simulink model "Edge_detector"  (Simulink 7.6)
settings: Solver=FixedStepDiscrete  SolverMode=SingleTasking  StartTime=0.0  StopTime=307201.0  RelTol=1e-3
InitFcn:
  | ed_in_script
  | %% DSPBuilder Start
  | alt_dspbuilder_update_model(bdroot)
  | %% DSPBuilder End
StopFcn:
  | ed_out_script
libraries: allblocks_alteradspbuilder2 x45
settings Model: Creator=lkong  LastModifiedBy=akarapet
settings DataIOCC: SignalLoggingName=sigsOut
settings OptimizationCC: InlineInvariantSignals=on  InitFltsAndDblsToZero=on
settings DebuggingCC: SaveWithParameterizedLinksMsg=none  SignalResolutionControl=TryResolveAllWithWarning  SolverPrmCheckMsg=none  MultiTaskDSMMsg=warning  MultiTaskCondExecSysMsg=none  StrictBusMsg=None
settings HardwareCC: TargetUnknown=on
settings RTWCC: IncludeERTFirstTime=on
settings GRTTargetCC: TargetFcnLib=ansi_tfl_tmw.mat

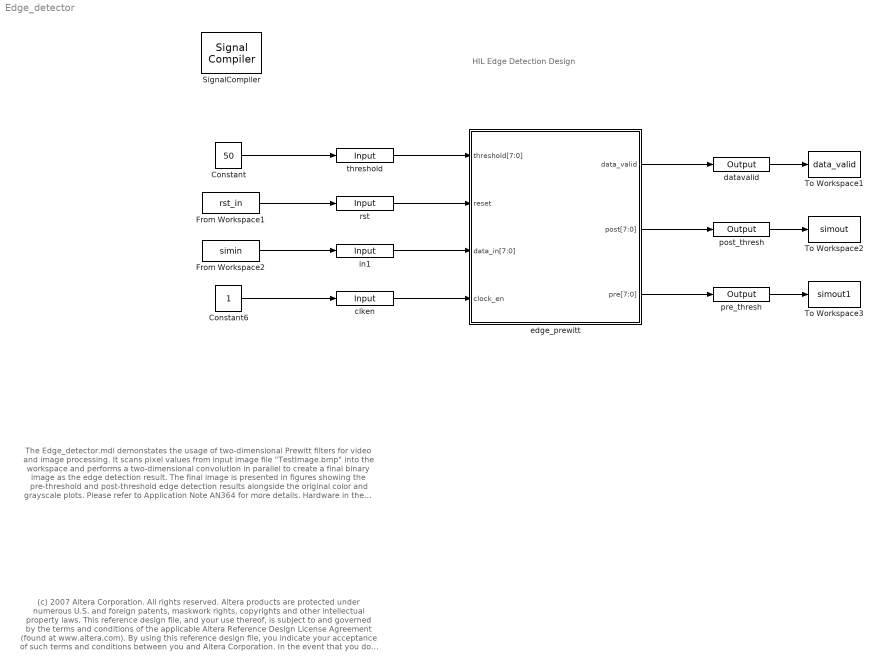
== system Edge_detector ==
  note: HIL Edge Detection Design
  note: The Edge_detector.mdl demonstates the usage of two-dimensional Prewitt filters for video and image processing.
      | It scans pixel values from input image file "TestImage.bmp" into the workspace and performs a two-dimensional
      | convolution in parallel to create a final binary image as the edge detection result.
      |
      | The final image is presented in figures showing the pre-threshold and post-threshold edge detection results
      | alongside the original color and grayscale plots.
      |
      | Please refer to Application Note AN364 for more details.
      |
      | Hardware in the Loop (HIL) is used to speed-up simulation as well as to verify the design in hardware.
  note: (c) 2007 Altera Corporation. All rights reserved.  Altera products are protected under numerous U.S. and foreign patents, maskwork rights, copyrights and other intellectual property laws.
      | This reference design file, and your use thereof, is subject to and governed by the terms and conditions of the applicable Altera Reference Design License Agreement (found at www.altera.com).
      | By using this reference design file, you indicate your acceptance of such terms and conditions between you and Altera Corporation.
      | In the event that you do not agree with such terms and conditions, you may not use the reference design file and please promptly destroy any copies you have made.
      | This reference design file being provided on an "as-is" basis and as an accommodation and therefore all warranties, representations or guarantees of any kind (whether express, implied or statutory)
      | including, without limitation, warranties of merchantability, non-infringement, or fitness for a particular purpose, are specifically disclaimed.
      | By making this reference design file available, Altera expressly does not recommend, suggest or require that this reference design file be used in combination with any other product not provided by Altera
  Constant : Constant  Value=50
  Constant6 : Constant
  From Workspace1 : FromWorkspace  VariableName=rst_in  SampleTime=1
  From Workspace2 : FromWorkspace  VariableName=simin  SampleTime=1
  SignalCompiler : allblocks_alteradspbuilder2/Signal Compiler  DeviceFamily=Cyclone III  DeviceName=EP3C120F780C7  EnableSignalTap=off  SignalTapDepth=1024  UseBoardBlock=off  StpUseDefaultClock=on  StpClock=Clock  ExportDir=/data/akarapet/qshell_linux64_test/p4/dsp_builder/dsp_builder2/Documentation/DesignExamples/Tutorials/HIL/EdgeDetection
  To Workspace1 : ToWorkspace  VariableName=data_valid  SaveFormat=Array
  To Workspace2 : ToWorkspace  VariableName=simout  SaveFormat=Array
  To Workspace3 : ToWorkspace  VariableName=simout1  SaveFormat=Array
  clken : allblocks_alteradspbuilder2/Input  iofile=/data/akarapet/qshell_linux64_test/p4/dsp_builder/dsp_builder2/Documentation/DesignExamples/Tutorials/HIL/EdgeDetection/tb_Edge_detector/Edge%5Fdetector_clken.salt  BusType=Single Bit  bwl=1  bwr=0  SpecifyClock=off  PORTTYPE=Input  externalType=Inferred  allowFloatingPointOverride=on  logOutputs=off
  datavalid : allblocks_alteradspbuilder2/Output  iofile=/data/akarapet/qshell_linux64_test/p4/dsp_builder/dsp_builder2/Documentation/DesignExamples/Tutorials/HIL/EdgeDetection/tb_Edge_detector/Edge%5Fdetector_datavalid.capture  BusType=Single Bit  bwl=1  bwr=0  externalType=Inferred  PORTTYPE=Output  allowFloatingPointOverride=on  logOutputs=off
  edge_prewitt : Subsystem
      mask Type: SubSystem AlteraBlockSet
  in1 : allblocks_alteradspbuilder2/Input  iofile=/data/akarapet/qshell_linux64_test/p4/dsp_builder/dsp_builder2/Documentation/DesignExamples/Tutorials/HIL/EdgeDetection/tb_Edge_detector/Edge%5Fdetector_in1.salt  BusType=Unsigned Integer  bwl=8  bwr=0  SpecifyClock=off  PORTTYPE=Input  externalType=Inferred  allowFloatingPointOverride=on  logOutputs=off
  post_thresh : allblocks_alteradspbuilder2/Output  iofile=/data/akarapet/qshell_linux64_test/p4/dsp_builder/dsp_builder2/Documentation/DesignExamples/Tutorials/HIL/EdgeDetection/tb_Edge_detector/Edge%5Fdetector_post%5Fthresh.capture  BusType=Unsigned Integer  bwl=8  bwr=0  externalType=Inferred  PORTTYPE=Output  allowFloatingPointOverride=on  logOutputs=off
  pre_thresh : allblocks_alteradspbuilder2/Output  iofile=/data/akarapet/qshell_linux64_test/p4/dsp_builder/dsp_builder2/Documentation/DesignExamples/Tutorials/HIL/EdgeDetection/tb_Edge_detector/Edge%5Fdetector_pre%5Fthresh.capture  BusType=Unsigned Integer  bwl=8  bwr=0  externalType=Inferred  PORTTYPE=Output  allowFloatingPointOverride=on  logOutputs=off
  rst : allblocks_alteradspbuilder2/Input  iofile=/data/akarapet/qshell_linux64_test/p4/dsp_builder/dsp_builder2/Documentation/DesignExamples/Tutorials/HIL/EdgeDetection/tb_Edge_detector/Edge%5Fdetector_rst.salt  BusType=Single Bit  bwl=1  bwr=0  SpecifyClock=off  PORTTYPE=Input  externalType=Inferred  allowFloatingPointOverride=on  logOutputs=off
  threshold : allblocks_alteradspbuilder2/Input  iofile=/data/akarapet/qshell_linux64_test/p4/dsp_builder/dsp_builder2/Documentation/DesignExamples/Tutorials/HIL/EdgeDetection/tb_Edge_detector/Edge%5Fdetector_threshold.salt  BusType=Unsigned Integer  bwl=8  bwr=0  SpecifyClock=off  PORTTYPE=Input  externalType=Inferred  allowFloatingPointOverride=on  logOutputs=off
  wires:
  Constant6/1 -> clken/1
  Constant/1 -> threshold/1
  From Workspace1/1 -> rst/1
  clken/1 -> edge_prewitt/4(clock_en)
  From Workspace2/1 -> in1/1
  in1/1 -> edge_prewitt/3(data_in[7:0])
  rst/1 -> edge_prewitt/2(reset)
  threshold/1 -> edge_prewitt/1(threshold[7:0])
  datavalid/1 -> To Workspace1/1
  edge_prewitt/2(post[7:0]) -> post_thresh/1
  edge_prewitt/1(data_valid) -> datavalid/1
  pre_thresh/1 -> To Workspace3/1
  post_thresh/1 -> To Workspace2/1
  edge_prewitt/3(pre[7:0]) -> pre_thresh/1

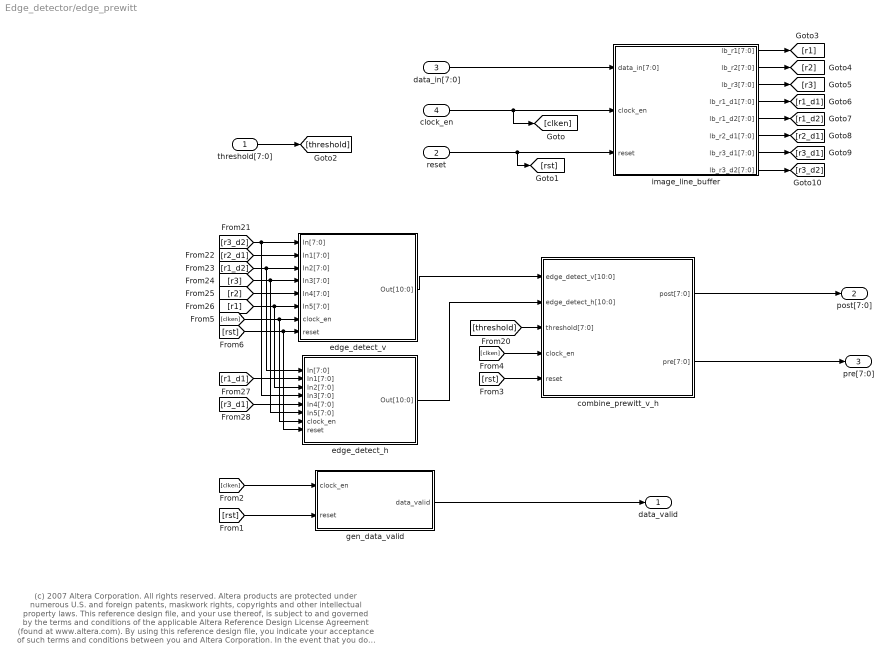
== system Edge_detector/edge_prewitt ==
  note: (c) 2007 Altera Corporation. All rights reserved.  Altera products are protected under numerous U.S. and foreign patents, maskwork rights, copyrights and other intellectual property laws.
      | This reference design file, and your use thereof, is subject to and governed by the terms and conditions of the applicable Altera Reference Design License Agreement (found at www.altera.com).
      | By using this reference design file, you indicate your acceptance of such terms and conditions between you and Altera Corporation.
      | In the event that you do not agree with such terms and conditions, you may not use the reference design file and please promptly destroy any copies you have made.
      | This reference design file being provided on an "as-is" basis and as an accommodation and therefore all warranties, representations or guarantees of any kind (whether express, implied or statutory)
      | including, without limitation, warranties of merchantability, non-infringement, or fitness for a particular purpose, are specifically disclaimed.
      | By making this reference design file available, Altera expressly does not recommend, suggest or require that this reference design file be used in combination with any other product not provided by Altera
  threshold[7:0] : Inport
  reset : Inport  Port=2
  data_in[7:0] : Inport  Port=3
  clock_en : Inport  Port=4
  combine_prewitt_v_h : Subsystem
      mask Type: SubSystem AlteraBlockSet
  edge_detect_h : Subsystem  AncestorBlock=ALTELINK/AltLab/HDL SubSystem
      mask Type: SubSystem AlteraBlockSet
  edge_detect_v : Subsystem  AncestorBlock=ALTELINK/AltLab/HDL SubSystem
      mask Type: SubSystem AlteraBlockSet
  gen_data_valid : Subsystem
      mask Type: SubSystem AlteraBlockSet
  image_line_buffer : Subsystem
      mask Type: SubSystem AlteraBlockSet
  data_valid : Outport
  post[7:0] : Outport  Port=2
  pre[7:0] : Outport  Port=3
  wires:
  edge_detect_v/1(Out[10:0]) -> combine_prewitt_v_h/1(edge_detect_v[10:0])
  edge_detect_h/1(Out[10:0]) -> combine_prewitt_v_h/2(edge_detect_h[10:0])
  [r3_d2] -> edge_detect_v/1(In[7:0]), edge_detect_h/4(In3[7:0])
  [r2_d1] -> edge_detect_v/2(In1[7:0])
  [r1_d2] -> edge_detect_v/3(In2[7:0]), edge_detect_h/1(In[7:0])
  [r3] -> edge_detect_v/4(In3[7:0]), edge_detect_h/6(In5[7:0])
  [r2] -> edge_detect_v/5(In4[7:0])
  [r1] -> edge_detect_v/6(In5[7:0]), edge_detect_h/3(In2[7:0])
  [r1_d1] -> edge_detect_h/2(In1[7:0])
  [r3_d1] -> edge_detect_h/5(In4[7:0])
  gen_data_valid/1(data_valid) -> data_valid/1
  image_line_buffer/1(lb_r1[7:0]) -> [r1]
  image_line_buffer/2(lb_r2[7:0]) -> [r2]
  image_line_buffer/3(lb_r3[7:0]) -> [r3]
  image_line_buffer/4(lb_r1_d1[7:0]) -> [r1_d1]
  image_line_buffer/5(lb_r1_d2[7:0]) -> [r1_d2]
  image_line_buffer/6(lb_r2_d1[7:0]) -> [r2_d1]
  image_line_buffer/7(lb_r3_d1[7:0]) -> [r3_d1]
  image_line_buffer/8(lb_r3_d2[7:0]) -> [r3_d2]
  [clken] -> gen_data_valid/1(clock_en)
  [rst] -> gen_data_valid/2(reset)
  [threshold] -> combine_prewitt_v_h/3(threshold[7:0])
  [clken] -> combine_prewitt_v_h/4(clock_en)
  [rst] -> combine_prewitt_v_h/5(reset)
  combine_prewitt_v_h/2(pre[7:0]) -> pre[7:0]/1
  combine_prewitt_v_h/1(post[7:0]) -> post[7:0]/1
  reset/1 -> image_line_buffer/3(reset), [rst]
  data_in[7:0]/1 -> image_line_buffer/1(data_in[7:0])
  clock_en/1 -> image_line_buffer/2(clock_en), [clken]
  [clken] -> edge_detect_v/7(clock_en), edge_detect_h/7(clock_en)
  [rst] -> edge_detect_v/8(reset), edge_detect_h/8(reset)
  threshold[7:0]/1 -> [threshold]

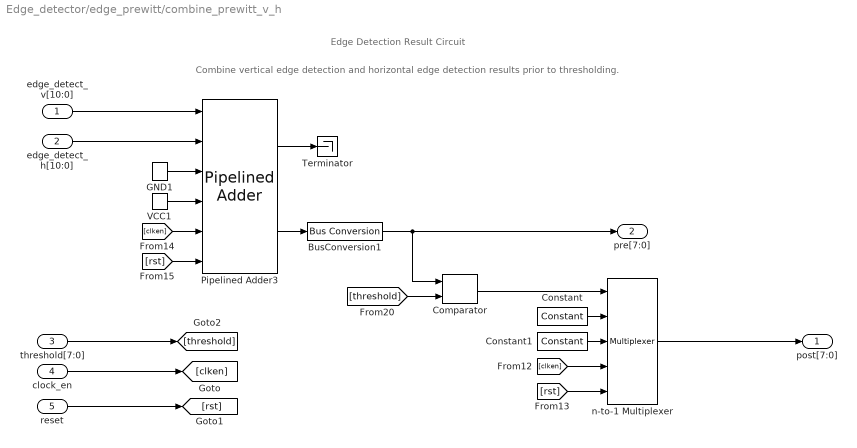
== system Edge_detector/edge_prewitt/combine_prewitt_v_h ==
  note: Combine vertical edge detection and horizontal edge detection results prior to thresholding.
  note: Edge Detection Result Circuit
  edge_detect_v[10:0] : Inport
  edge_detect_h[10:0] : Inport  Port=2
  threshold[7:0] : Inport  Port=3
  clock_en : Inport  Port=4
  reset : Inport  Port=5
  BusConversion1 : allblocks_alteradspbuilder2/Bus Conversion  BusType=Unsigned Integer  ibwl=11  ibwr=0  bwl=8  bwr=0  bitToConnectToOutputLSB=0  round=off  saturate=on  pipeline_display=0
  Comparator : allblocks_alteradspbuilder2/Comparator  direction=a < b  pipeline_display=0  allowFloatingPointOverride=on  logOutputs=off  logFile=/data/akarapet/qshell_linux64_test/p4/dsp_builder/dsp_builder2/Documentation/DesignExamples/Tutorials/HIL/EdgeDetection/tb_Edge_detector/Edge%5Fdetector_edge%5Fprewitt_combine%5Fprewitt%5Fv%5Fh_Comparator.fixedpointlog
  Constant : allblocks_alteradspbuilder2/Constant  mask_cst=255  BusType=Unsigned Integer  bwl=8  bwr=0  roundMode=Truncate  satMode=Wrap  SpecifyClock=off  allowFloatingPointOverride=on  logOutputs=off  logFile=/data/akarapet/qshell_linux64_test/p4/dsp_builder/dsp_builder2/Documentation/DesignExamples/Tutorials/HIL/EdgeDetection/tb_Edge_detector/Edge%5Fdetector_edge%5Fprewitt_combine%5Fprewitt%5Fv%5Fh_Constant.fixedpointlog
  Constant1 : allblocks_alteradspbuilder2/Constant  mask_cst=0  BusType=Unsigned Integer  bwl=8  bwr=0  roundMode=Truncate  satMode=Wrap  SpecifyClock=off  allowFloatingPointOverride=on  logOutputs=off  logFile=/data/akarapet/qshell_linux64_test/p4/dsp_builder/dsp_builder2/Documentation/DesignExamples/Tutorials/HIL/EdgeDetection/tb_Edge_detector/Edge%5Fdetector_edge%5Fprewitt_combine%5Fprewitt%5Fv%5Fh_Constant1.fixedpointlog
  GND1 : allblocks_alteradspbuilder2/GND  SpecifyClock=off
  Pipelined Adder3 : allblocks_alteradspbuilder2/Pipelined Adder  BusType=Unsigned Integer  bwl=11  bwr=0  pipeline=1  pipeline_display=1  AddSubDirection=ADD  use_cin=on  use_ovl=on  use_addsub=on  use_ena=on  use_aclr=on  or_aclr_inputs=on
  Terminator : Terminator
  VCC1 : allblocks_alteradspbuilder2/VCC  SpecifyClock=off
  n-to-1 Multiplexer : allblocks_alteradspbuilder2/Multiplexer  numInputs=2  pipeline=1  oneHot=off  pipeline_display=1  use_ena=on  use_aclr=on  allowFloatingPointOverride=on  logOutputs=off  logFile=/data/akarapet/qshell_linux64_test/p4/dsp_builder/dsp_builder2/Documentation/DesignExamples/Tutorials/HIL/EdgeDetection/tb_Edge_detector/Edge%5Fdetector_edge%5Fprewitt_combine%5Fprewitt%5Fv%5Fh_n-to-1+Multiplexer.fixedpointlog
  post[7:0] : Outport
  pre[7:0] : Outport  Port=2
  wires:
  Comparator/1 -> n-to-1 Multiplexer/1
  Constant/1 -> n-to-1 Multiplexer/2
  Constant1/1 -> n-to-1 Multiplexer/3
  BusConversion1/1 -> Comparator/1, pre[7:0]/1
  [clken] -> n-to-1 Multiplexer/4
  [rst] -> n-to-1 Multiplexer/5
  Pipelined Adder3/2 -> BusConversion1/1
  GND1/1 -> Pipelined Adder3/3
  VCC1/1 -> Pipelined Adder3/4
  [clken] -> Pipelined Adder3/5
  [rst] -> Pipelined Adder3/6
  edge_detect_v[10:0]/1 -> Pipelined Adder3/1
  edge_detect_h[10:0]/1 -> Pipelined Adder3/2
  threshold[7:0]/1 -> [threshold]
  reset/1 -> [rst]
  n-to-1 Multiplexer/1 -> post[7:0]/1
  clock_en/1 -> [clken]
  [threshold] -> Comparator/2
  Pipelined Adder3/1 -> Terminator/1

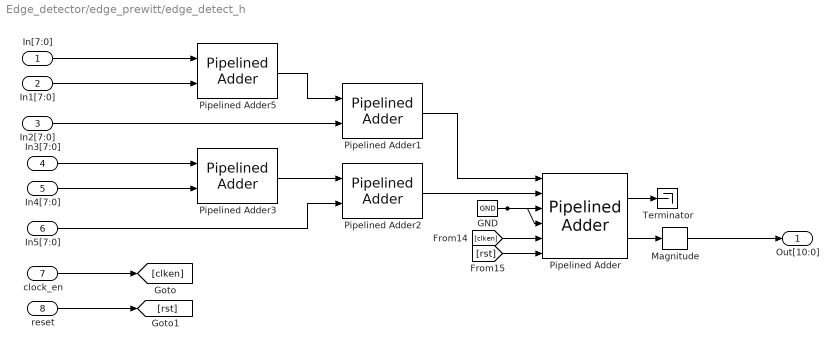
== system Edge_detector/edge_prewitt/edge_detect_h ==
  In[7:0] : Inport
  In1[7:0] : Inport  Port=2
  In2[7:0] : Inport  Port=3
  In3[7:0] : Inport  Port=4
  In4[7:0] : Inport  Port=5
  In5[7:0] : Inport  Port=6
  clock_en : Inport  Port=7
  reset : Inport  Port=8
  GND : allblocks_alteradspbuilder2/GND  SpecifyClock=off
  Magnitude : allblocks_alteradspbuilder2/Magnitude  pipeline_display=0
  Pipelined Adder : allblocks_alteradspbuilder2/Pipelined Adder  BusType=Signed Integer  bwl=11  bwr=0  pipeline=1  pipeline_display=1  AddSubDirection=ADD  use_cin=on  use_ovl=on  use_addsub=on  use_ena=on  use_aclr=on  or_aclr_inputs=on
  Pipelined Adder1 : allblocks_alteradspbuilder2/Pipelined Adder  BusType=Unsigned Integer  bwl=10  bwr=0  pipeline=0  pipeline_display=0  AddSubDirection=ADD  use_cin=off  use_ovl=off  use_addsub=off  use_ena=off  use_aclr=off  or_aclr_inputs=on
  Pipelined Adder2 : allblocks_alteradspbuilder2/Pipelined Adder  BusType=Unsigned Integer  bwl=10  bwr=0  pipeline=0  pipeline_display=0  AddSubDirection=ADD  use_cin=off  use_ovl=off  use_addsub=off  use_ena=off  use_aclr=off  or_aclr_inputs=on
  Pipelined Adder3 : allblocks_alteradspbuilder2/Pipelined Adder  BusType=Unsigned Integer  bwl=9  bwr=0  pipeline=0  pipeline_display=0  AddSubDirection=ADD  use_cin=off  use_ovl=off  use_addsub=off  use_ena=off  use_aclr=off  or_aclr_inputs=on
  Pipelined Adder5 : allblocks_alteradspbuilder2/Pipelined Adder  BusType=Unsigned Integer  bwl=9  bwr=0  pipeline=0  pipeline_display=0  AddSubDirection=ADD  use_cin=off  use_ovl=off  use_addsub=off  use_ena=off  use_aclr=off  or_aclr_inputs=on
  Terminator : Terminator
  Out[10:0] : Outport
  wires:
  In[7:0]/1 -> Pipelined Adder5/1
  In1[7:0]/1 -> Pipelined Adder5/2
  In2[7:0]/1 -> Pipelined Adder1/2
  Pipelined Adder5/1 -> Pipelined Adder1/1
  In3[7:0]/1 -> Pipelined Adder3/1
  In4[7:0]/1 -> Pipelined Adder3/2
  Pipelined Adder3/1 -> Pipelined Adder2/1
  Pipelined Adder1/1 -> Pipelined Adder/1
  Pipelined Adder2/1 -> Pipelined Adder/2
  Magnitude/1 -> Out[10:0]/1
  GND/1 -> Pipelined Adder/3, Pipelined Adder/4
  In5[7:0]/1 -> Pipelined Adder2/2
  reset/1 -> [rst]
  clock_en/1 -> [clken]
  Pipelined Adder/2 -> Magnitude/1
  [clken] -> Pipelined Adder/5
  [rst] -> Pipelined Adder/6
  Pipelined Adder/1 -> Terminator/1

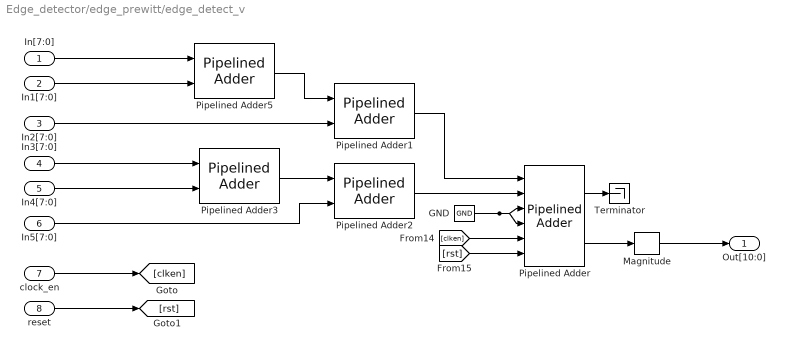
== system Edge_detector/edge_prewitt/edge_detect_v ==
  In[7:0] : Inport
  In1[7:0] : Inport  Port=2
  In2[7:0] : Inport  Port=3
  In3[7:0] : Inport  Port=4
  In4[7:0] : Inport  Port=5
  In5[7:0] : Inport  Port=6
  clock_en : Inport  Port=7
  reset : Inport  Port=8
  GND : allblocks_alteradspbuilder2/GND  SpecifyClock=off
  Magnitude : allblocks_alteradspbuilder2/Magnitude  pipeline_display=0
  Pipelined Adder : allblocks_alteradspbuilder2/Pipelined Adder  BusType=Signed Integer  bwl=11  bwr=0  pipeline=1  pipeline_display=1  AddSubDirection=ADD  use_cin=on  use_ovl=on  use_addsub=on  use_ena=on  use_aclr=on  or_aclr_inputs=on
  Pipelined Adder1 : allblocks_alteradspbuilder2/Pipelined Adder  BusType=Unsigned Integer  bwl=10  bwr=0  pipeline=0  pipeline_display=0  AddSubDirection=ADD  use_cin=off  use_ovl=off  use_addsub=off  use_ena=off  use_aclr=off  or_aclr_inputs=on
  Pipelined Adder2 : allblocks_alteradspbuilder2/Pipelined Adder  BusType=Unsigned Integer  bwl=10  bwr=0  pipeline=0  pipeline_display=0  AddSubDirection=ADD  use_cin=off  use_ovl=off  use_addsub=off  use_ena=off  use_aclr=off  or_aclr_inputs=on
  Pipelined Adder3 : allblocks_alteradspbuilder2/Pipelined Adder  BusType=Unsigned Integer  bwl=9  bwr=0  pipeline=0  pipeline_display=0  AddSubDirection=ADD  use_cin=off  use_ovl=off  use_addsub=off  use_ena=off  use_aclr=off  or_aclr_inputs=on
  Pipelined Adder5 : allblocks_alteradspbuilder2/Pipelined Adder  BusType=Unsigned Integer  bwl=9  bwr=0  pipeline=0  pipeline_display=0  AddSubDirection=ADD  use_cin=off  use_ovl=off  use_addsub=off  use_ena=off  use_aclr=off  or_aclr_inputs=on
  Terminator : Terminator
  Out[10:0] : Outport
  wires:
  In[7:0]/1 -> Pipelined Adder5/1
  In1[7:0]/1 -> Pipelined Adder5/2
  In2[7:0]/1 -> Pipelined Adder1/2
  Pipelined Adder5/1 -> Pipelined Adder1/1
  In3[7:0]/1 -> Pipelined Adder3/1
  In4[7:0]/1 -> Pipelined Adder3/2
  In5[7:0]/1 -> Pipelined Adder2/2
  Pipelined Adder3/1 -> Pipelined Adder2/1
  Pipelined Adder1/1 -> Pipelined Adder/1
  Pipelined Adder2/1 -> Pipelined Adder/2
  Magnitude/1 -> Out[10:0]/1
  GND/1 -> Pipelined Adder/3, Pipelined Adder/4
  Pipelined Adder/2 -> Magnitude/1
  reset/1 -> [rst]
  clock_en/1 -> [clken]
  [clken] -> Pipelined Adder/5
  [rst] -> Pipelined Adder/6
  Pipelined Adder/1 -> Terminator/1

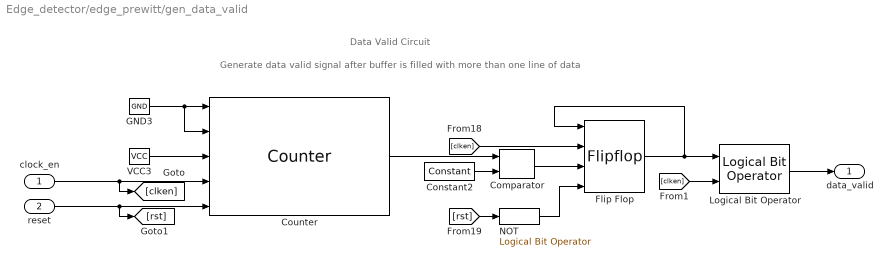
== system Edge_detector/edge_prewitt/gen_data_valid ==
  note: Generate data valid signal after buffer is filled with more than one line of data
  note: Data Valid Circuit
  clock_en : Inport
  reset : Inport  Port=2
  Comparator : allblocks_alteradspbuilder2/Comparator  direction=a < b  pipeline_display=0  allowFloatingPointOverride=on  logOutputs=off  logFile=/data/akarapet/qshell_linux64_test/p4/dsp_builder/dsp_builder2/Documentation/DesignExamples/Tutorials/HIL/EdgeDetection/tb_Edge_detector/Edge%5Fdetector_edge%5Fprewitt_gen%5Fdata%5Fvalid_Comparator.fixedpointlog
  Constant2 : allblocks_alteradspbuilder2/Constant  mask_cst=640+3  BusType=Unsigned Integer  bwl=12  bwr=0  roundMode=Truncate  satMode=Wrap  SpecifyClock=off  allowFloatingPointOverride=on  logOutputs=off  logFile=/data/akarapet/qshell_linux64_test/p4/dsp_builder/dsp_builder2/Documentation/DesignExamples/Tutorials/HIL/EdgeDetection/tb_Edge_detector/Edge%5Fdetector_edge%5Fprewitt_gen%5Fdata%5Fvalid_Constant2.fixedpointlog
  Counter : allblocks_alteradspbuilder2/Counter  BusType=Unsigned Integer  bwl=13  bwr=0  use_modulo=on  modulo=8*640  SpecifyClock=off  direction=Use Direction Port (updown)  use_sload=on  use_sset=off  svalue=1  use_clk_ena=off  use_ena=on  use_sclr=on  pipeline_display=1
  Flip Flop : allblocks_alteradspbuilder2/Flipflop  mode=DFFE  BusType=Signed Fractional  bwl=1  bwr=1  pipeline_display=1
  GND3 : allblocks_alteradspbuilder2/GND  SpecifyClock=off
  Logical Bit Operator : allblocks_alteradspbuilder2/Logical Bit Operator  LogicalOperator=AND  user_inputs=2  pipeline_display=0
  NOT : allblocks_alteradspbuilder2/Logical Bit Operator  LogicalOperator=NOT  user_inputs=2  pipeline_display=0
  VCC3 : allblocks_alteradspbuilder2/VCC  SpecifyClock=off
  data_valid : Outport
  wires:
  Counter/1 -> Comparator/1
  Comparator/1 -> Flip Flop/3
  [clken] -> Flip Flop/2
  NOT/1 -> Flip Flop/4
  [rst] -> NOT/1
  Flip Flop/1 -> Flip Flop/1, Logical Bit Operator/1
  Constant2/1 -> Comparator/2
  VCC3/1 -> Counter/3
  clock_en/1 -> Counter/4, [clken]
  reset/1 -> Counter/5, [rst]
  Logical Bit Operator/1 -> data_valid/1
  [clken] -> Logical Bit Operator/2
  GND3/1 -> Counter/1, Counter/2

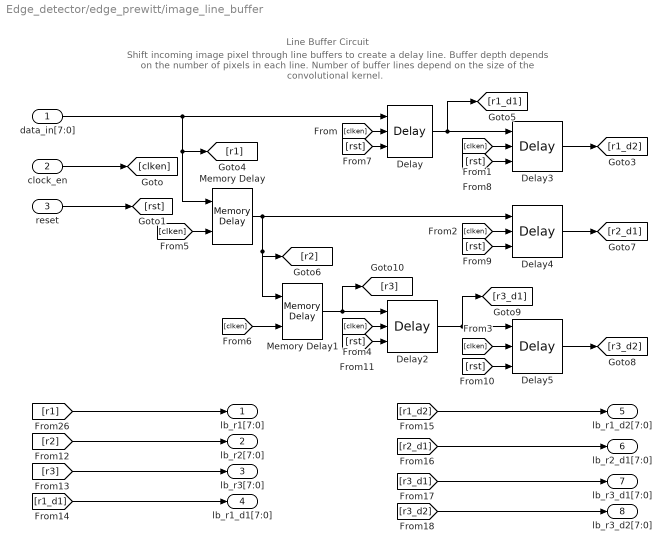
== system Edge_detector/edge_prewitt/image_line_buffer ==
  note: Shift incoming image pixel through line buffers to create a delay line.  Buffer depth depends on the number of pixels
      | in each line.  Number of buffer lines depend on the size of the convolutional kernel.
  note: Line Buffer Circuit
  data_in[7:0] : Inport
  clock_en : Inport  Port=2
  reset : Inport  Port=3
  Delay : allblocks_alteradspbuilder2/Delay  pipeline=1  pipeline_display=1  ClockPhase=1  use_ena=on  use_sclr=on  allowFloatingPointOverride=on  logOutputs=off  logFile=/data/akarapet/qshell_linux64_test/p4/dsp_builder/dsp_builder2/Documentation/DesignExamples/Tutorials/HIL/EdgeDetection/tb_Edge_detector/Edge%5Fdetector_edge%5Fprewitt_image%5Fline%5Fbuffer_Delay.fixedpointlog  use_init=off  reset_value=1
  Delay2 : allblocks_alteradspbuilder2/Delay  pipeline=1  pipeline_display=1  ClockPhase=1  use_ena=on  use_sclr=on  allowFloatingPointOverride=on  logOutputs=off  logFile=/data/akarapet/qshell_linux64_test/p4/dsp_builder/dsp_builder2/Documentation/DesignExamples/Tutorials/HIL/EdgeDetection/tb_Edge_detector/Edge%5Fdetector_edge%5Fprewitt_image%5Fline%5Fbuffer_Delay2.fixedpointlog  use_init=off  reset_value=1
  Delay3 : allblocks_alteradspbuilder2/Delay  pipeline=1  pipeline_display=1  ClockPhase=1  use_ena=on  use_sclr=on  allowFloatingPointOverride=on  logOutputs=off  logFile=/data/akarapet/qshell_linux64_test/p4/dsp_builder/dsp_builder2/Documentation/DesignExamples/Tutorials/HIL/EdgeDetection/tb_Edge_detector/Edge%5Fdetector_edge%5Fprewitt_image%5Fline%5Fbuffer_Delay3.fixedpointlog  use_init=off  reset_value=1
  Delay4 : allblocks_alteradspbuilder2/Delay  pipeline=2  pipeline_display=2  ClockPhase=1  use_ena=on  use_sclr=on  allowFloatingPointOverride=on  logOutputs=off  logFile=/data/akarapet/qshell_linux64_test/p4/dsp_builder/dsp_builder2/Documentation/DesignExamples/Tutorials/HIL/EdgeDetection/tb_Edge_detector/Edge%5Fdetector_edge%5Fprewitt_image%5Fline%5Fbuffer_Delay4.fixedpointlog  use_init=off  reset_value=1
  Delay5 : allblocks_alteradspbuilder2/Delay  pipeline=1  pipeline_display=1  ClockPhase=1  use_ena=on  use_sclr=on  allowFloatingPointOverride=on  logOutputs=off  logFile=/data/akarapet/qshell_linux64_test/p4/dsp_builder/dsp_builder2/Documentation/DesignExamples/Tutorials/HIL/EdgeDetection/tb_Edge_detector/Edge%5Fdetector_edge%5Fprewitt_image%5Fline%5Fbuffer_Delay5.fixedpointlog  use_init=off  reset_value=1
  Memory Delay : allblocks_alteradspbuilder2/Memory Delay  BusType=Inferred  bwl=8  bwr=0  pipeline=640  pipeline_display=640  ram_type=AUTO  use_ena=on  use_sclr=off  allowFloatingPointOverride=on  logOutputs=off  logFile=/data/akarapet/qshell_linux64_test/p4/dsp_builder/dsp_builder2/Documentation/DesignExamples/Tutorials/HIL/EdgeDetection/tb_Edge_detector/Edge%5Fdetector_edge%5Fprewitt_image%5Fline%5Fbuffer_Memory+Delay.fixedpointlog
  Memory Delay1 : allblocks_alteradspbuilder2/Memory Delay  BusType=Inferred  bwl=8  bwr=0  pipeline=640  pipeline_display=640  ram_type=AUTO  use_ena=on  use_sclr=off  allowFloatingPointOverride=on  logOutputs=off  logFile=/data/akarapet/qshell_linux64_test/p4/dsp_builder/dsp_builder2/Documentation/DesignExamples/Tutorials/HIL/EdgeDetection/tb_Edge_detector/Edge%5Fdetector_edge%5Fprewitt_image%5Fline%5Fbuffer_Memory+Delay1.fixedpointlog
  lb_r1[7:0] : Outport
  lb_r2[7:0] : Outport  Port=2
  lb_r3[7:0] : Outport  Port=3
  lb_r1_d1[7:0] : Outport  Port=4
  lb_r1_d2[7:0] : Outport  Port=5
  lb_r2_d1[7:0] : Outport  Port=6
  lb_r3_d1[7:0] : Outport  Port=7
  lb_r3_d2[7:0] : Outport  Port=8
  wires:
  Memory Delay/1 -> Delay4/1, Memory Delay1/1, [r2]
  Memory Delay1/1 -> Delay2/1, [r3]
  [clken] -> Delay/2
  [clken] -> Delay3/2
  [clken] -> Delay4/2
  [clken] -> Delay5/2
  [clken] -> Delay2/2
  [clken] -> Memory Delay/2
  [clken] -> Memory Delay1/2
  [rst] -> Delay/3
  [rst] -> Delay3/3
  [rst] -> Delay2/3
  [rst] -> Delay4/3
  [rst] -> Delay5/3
  Delay/1 -> Delay3/1, [r1_d1]
  Delay2/1 -> Delay5/1, [r3_d1]
  data_in[7:0]/1 -> [r1], Memory Delay/1, Delay/1
  Delay3/1 -> [r1_d2]
  Delay4/1 -> [r2_d1]
  Delay5/1 -> [r3_d2]
  clock_en/1 -> [clken]
  reset/1 -> [rst]
  [r1] -> lb_r1[7:0]/1
  [r2] -> lb_r2[7:0]/1
  [r3] -> lb_r3[7:0]/1
  [r1_d1] -> lb_r1_d1[7:0]/1
  [r1_d2] -> lb_r1_d2[7:0]/1
  [r2_d1] -> lb_r2_d1[7:0]/1
  [r3_d1] -> lb_r3_d1[7:0]/1
  [r3_d2] -> lb_r3_d2[7:0]/1
